simulink model "es5"  (R2022b)
settings: Solver=VariableStepAuto  StartTime=0.0  StopTime=10  RelTol=1e-3
settings Model: Creator=adlercohen  LastModifiedBy=adlercohen
settings DataIOCC: ReturnWorkspaceOutputs=off

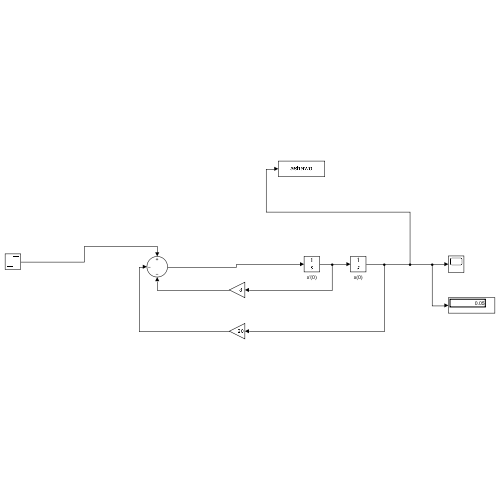
[thumbnail: Simulink's stored preview of the top-level diagram]
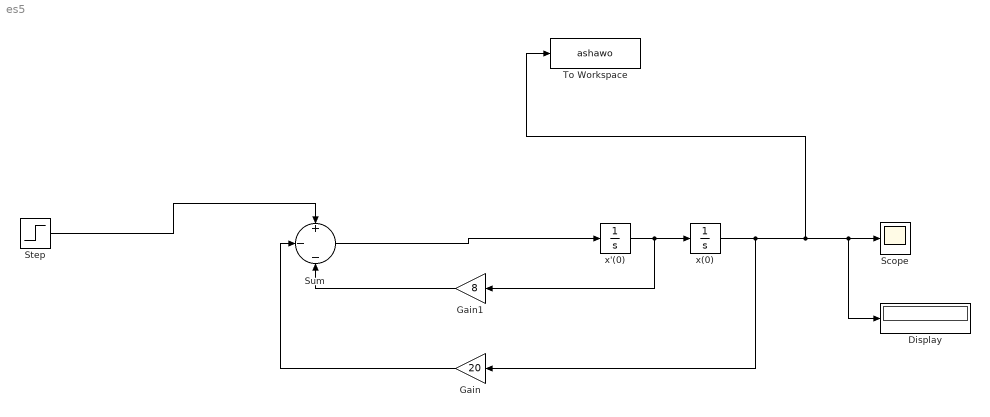
== system es5 ==
  Display : Display
  Gain : Gain  Gain=20
  Gain1 : Gain  Gain=8
  Scope : Scope
  Step : Step  Time=0  SampleTime=0
  Sum : Sum  Inputs=+|-|-
  To Workspace : ToWorkspace  VariableName=ashawo  SampleTime=-1
  x'(0) : Integrator  InitialCondition=0.5
  x(0) : Integrator
  wires:
  x'(0)/1 -> Gain1/1, x(0)/1
  Gain/1 -> Sum/2
  Gain1/1 -> Sum/3
  Step/1 -> Sum/1
  x(0)/1 -> To Workspace/1, Scope/1, Display/1, Gain/1
  Sum/1 -> x'(0)/1
